simulink model "P_CGMRES_fast"  (R2023a)
settings: Solver=FixedStepAuto  StartTime=0.0  StopTime=22.16  RelTol=1e-3
values from neighbouring files (symbols this model uses):
  lujing = 8    [main.m]
libraries: Solver_SF x1
(part 1 of 21)
settings Model: Creator=Administrator  LastModifiedBy=Lenovo
settings SolverCC: AlgebraicLoopSolver=TrustRegion
settings OptimizationCC: LifeSpan=inf
settings DebuggingCC: UnconnectedInputMsg=warning  UnconnectedOutputMsg=warning  UnconnectedLineMsg=warning  ArithmeticOperatorsInVariantConditions=warning
settings ModelReferenceCC: EnableRefExpFcnMdlSchedulingChecks=on
settings SFSimCC: CustomCodeUndefinedFunction=UseInterfaceOnly
settings CodeAppCC: StateflowObjectComments=on

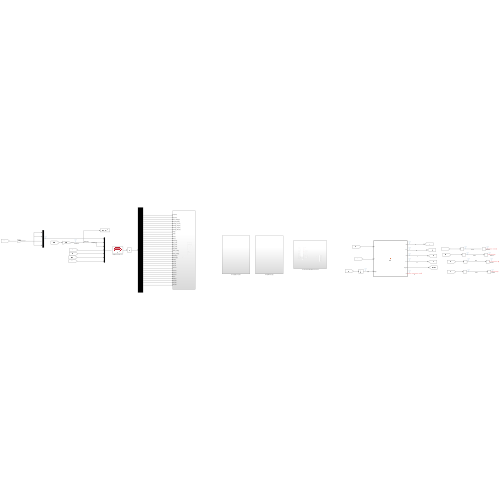
[thumbnail: Simulink's stored preview of the top-level diagram]
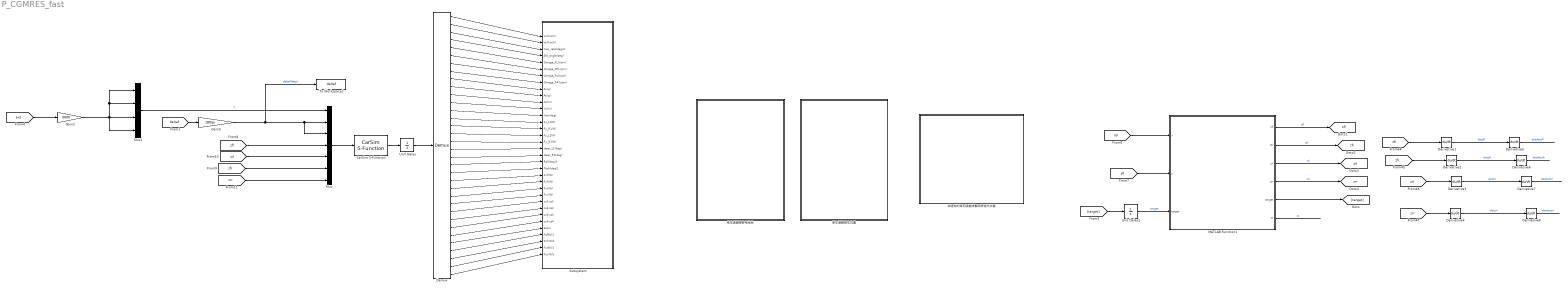
== system P_CGMRES_fast ==
  CarSim S-Function : Solver_SF/CarSim S-Function  Priority=1  SIMFILE=simfile.sim  Run_RTs=off  vs_state_ind=Run  StopMode_ind=Vehicle Model
  Demux : Demux  Outputs=34
  Derivative{1..8} (8 alike) : Derivative
  Gain2 : Gain  Gain=3000
  Gain3 : Gain  Gain=180/pi
  MATLAB Function1 : MATLAB Function  TreatAsAtomicUnit=on
  Mux : Mux  Inputs=7
  Mux1 : Mux
  Subsystem : Subsystem
  To Workspace2 : ToWorkspace  VariableName=deltaf  SaveFormat=Timeseries  SampleTime=-1
  Unit Delay : UnitDelay  InitialCondition=[50,0.01*ones(1,24),0,0,0,0,0,3575,3575,3575,3575]  SampleTime=-1  HasFrameUpgradeWarning=on
  Unit Delay1 : UnitDelay  InitialCondition=1  SampleTime=-1  HasFrameUpgradeWarning=on
  单车道避障参考坐标 : Subsystem
  单车道障碍车位置 : Subsystem
  快速有约束罚函数求解同样迭代次数 : Subsystem
  tag scope: zfl=global, zfr=global, zrl=global, zrr=global
  wires:
  Unit Delay/1 -> Demux/1
  Demux/1 -> Subsystem/1(Vx(km/h))
  Demux/2 -> Subsystem/2(Vy(km/h))
  Demux/3 -> Subsystem/3(Yaw_rate(deg/s))
  Demux/4 -> Subsystem/4(SW_angle(deg))
  Demux/5 -> Subsystem/5(Omega_FL(r/pm))
  Demux/6 -> Subsystem/6(Omega_FR(r/pm))
  Demux/7 -> Subsystem/7(Omega_RL(r/pm))
  Demux/8 -> Subsystem/8(Omega_RR(r/pm))
  Demux/9 -> Subsystem/9(Ax(g))
  Demux/10 -> Subsystem/10(Ay(g))
  Demux/11 -> Subsystem/11(Xo(m))
  Demux/12 -> Subsystem/12(Yo(m))
  Demux/13 -> Subsystem/13(Yaw(deg))
  Demux/14 -> Subsystem/14(Fy_L1(N))
  Demux/15 -> Subsystem/15(Fy_R1(N))
  Demux/16 -> Subsystem/16(Fy_L2(N))
  Demux/17 -> Subsystem/17(Fy_R2(N))
  Demux/18 -> Subsystem/18(steer_L1(deg))
  Demux/19 -> Subsystem/19(steer_R1(deg))
  Mux/1 -> CarSim S-Function/1
  CarSim S-Function/1 -> Unit Delay/1
  [ax2] -> Gain2/1
  Gain2/1 -> Mux1/4, Mux1/3, Mux1/2, Mux1/1
  Mux1/1 -> Mux/1  "T"
  [deltaf] -> Gain3/1
  [zfl] -> Mux/4
  Demux/20 -> Subsystem/20(Roll(deg)1)
  Demux/21 -> Subsystem/21(Pitch(deg)1)
  [zrl] -> Mux/5
  [zfr] -> Mux/6
  [zrr] -> Mux/7
  Demux/22 -> Subsystem/22(Fxfl(N))
  Demux/23 -> Subsystem/23(Fxfr(N))
  Demux/24 -> Subsystem/24(Fxrl(N))
  Demux/25 -> Subsystem/25(Fxrr(N))
  Demux/26 -> Subsystem/26(zu1-zs1)
  Demux/27 -> Subsystem/27(zu2-zs2)
  Demux/28 -> Subsystem/28(zu3-zs3)
  Demux/29 -> Subsystem/29(zu4-zs4)
  Demux/30 -> Subsystem/30(azsm)
  Demux/31 -> Subsystem/31(Fzfl(N)1)
  Demux/32 -> Subsystem/32(Fzfr(N)1)
  Demux/33 -> Subsystem/33(Fzrl(N)1)
  Demux/34 -> Subsystem/34(Fzrr(N)1)
  MATLAB Function1/3(zrl) -> [zrl]  "zrl"
  [zfr] -> Derivative2/1
  Derivative2/1 -> Derivative6/1  "dotzfr"
  Unit Delay1/1 -> MATLAB Function1/3("target ")  "target"
  [target] -> Unit Delay1/1
  [y0] -> MATLAB Function1/2(y)
  [zrr] -> Derivative4/1
  [zfl] -> Derivative1/1
  MATLAB Function1/1(zfl) -> [zfl]  "zfl"
  Derivative1/1 -> Derivative5/1  "dotzfl"
  [zrl] -> Derivative3/1
  Derivative4/1 -> Derivative8/1  "dotzrr"
  MATLAB Function1/4(zrr) -> [zrr]  "zrr"
  [x0] -> MATLAB Function1/1(x)
  MATLAB Function1/5(target) -> [target]
  Derivative3/1 -> Derivative7/1  "dotzrl"
  Derivative6/1 -> ?  "dotdotzfr"
  MATLAB Function1/2(zfr) -> [zfr]  "zfr"
  Derivative5/1 -> ?  "dotdotzfl"
  MATLAB Function1/6(zz) -> ?  "zz"
  Derivative8/1 -> ?  "dotdotzrr"
  Derivative7/1 -> ?  "dotdotzrl"
  Gain3/1 -> To Workspace2/1, Mux/3, Mux/2  "deltaf(deg)"

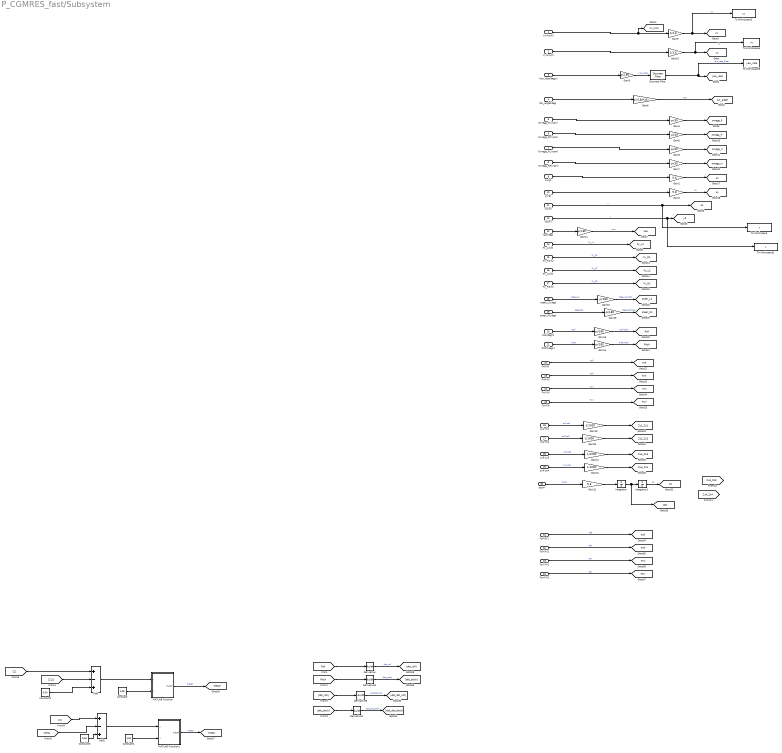
== system P_CGMRES_fast/Subsystem ==
  Vx(km/h) : Inport
  Vy(km/h) : Inport  Port=2
  Yaw_rate(deg/s) : Inport  Port=3
  SW_angle(deg) : Inport  Port=4
  Omega_FL(r/pm) : Inport  Port=5
  Omega_FR(r/pm) : Inport  Port=6
  Omega_RL(r/pm) : Inport  Port=7
  Omega_RR(r/pm) : Inport  Port=8
  Ax(g) : Inport  Port=9
  Ay(g) : Inport  Port=10
  Xo(m) : Inport  Port=11
  Yo(m) : Inport  Port=12
  Yaw(deg) : Inport  Port=13
  Fy_L1(N) : Inport  Port=14
  Fy_R1(N) : Inport  Port=15
  Fy_L2(N) : Inport  Port=16
  Fy_R2(N) : Inport  Port=17
  steer_L1(deg) : Inport  Port=18
  steer_R1(deg) : Inport  Port=19
  Roll(deg)1 : Inport  Port=20
  Pitch(deg)1 : Inport  Port=21
  Fxfl(N) : Inport  Port=22
  Fxfr(N) : Inport  Port=23
  Fxrl(N) : Inport  Port=24
  Fxrr(N) : Inport  Port=25
  zu1-zs1 : Inport  Port=26
  zu2-zs2 : Inport  Port=27
  zu3-zs3 : Inport  Port=28
  zu4-zs4 : Inport  Port=29
  azsm : Inport  Port=30
  Fzfl(N)1 : Inport  Port=31
  Fzfr(N)1 : Inport  Port=32
  Fzrl(N)1 : Inport  Port=33
  Fzrr(N)1 : Inport  Port=34
  Add : Sum  Inputs=+-+
  Add1 : Sum  Inputs=+-+
  Constant : Constant  Value=1.05
  Constant1 : Constant  Value=1.61
  Constant2 : Constant  Value=0.54
  Constant3 : Constant  Value=0.54
  Derivative{,1..3} (4 alike) : Derivative
  Discrete Filter : DiscreteFilter
  Gain1 : Gain  Gain=9.8
  Gain10 : Gain  Gain=1/3.6
  Gain{3,11,13..16} (6 alike) : Gain  Gain=pi/180
  Gain12 : Gain  Gain=9.8
  Gain{19..22} (4 alike) : Gain  Gain=1/1000
  Gain2 : Gain  Gain=9.8
  Gain{4..7} (4 alike) : Gain  Gain=pi/30
  Gain8 : Gain  Gain=pi/(180*16)
  Gain9 : Gain  Gain=1/3.6
  Integrator : Integrator
  Integrator1 : Integrator  InitialCondition=0.54
  MATLAB Function : MATLAB Function  TreatAsAtomicUnit=on
  MATLAB Function1 : MATLAB Function  TreatAsAtomicUnit=on
  To Workspace : ToWorkspace  VariableName=x  SaveFormat=Timeseries  SampleTime=-1
  To Workspace1 : ToWorkspace  VariableName=y  SaveFormat=Timeseries  SampleTime=-1
  To Workspace2 : ToWorkspace  VariableName=vx  SaveFormat=Timeseries  SampleTime=-1
  To Workspace3 : ToWorkspace  VariableName=yaw_rate  SampleTime=-1
      settings: Save2DSignal=2-D array (concatenate along first dimension)
  To Workspace4 : ToWorkspace  VariableName=Vy  SampleTime=-1
      settings: Save2DSignal=2-D array (concatenate along first dimension)
  tag scope: Fxfl=global, Fxfr=global, Fxrl=global, Fxrr=global, Fy_L1=global, Fy_L2=global, Fy_R1=global, Fy_R2=global, Fzfl=global, Fzfr=global, Fzrl=global, Fzrr=global, Pitch=global, Roll=global, Vx=global, Vx_kmh=global, Vy=global, Yaw=global, Zs=global, Zu1_Zs1=global, Zu2_Zs2=global, Zu3_Zs3=global, Zu4_Zs4=global, ax=global, ay=global, dZs=global, omega_fl=global, omega_fr=global, omega_rl=global, omega_rr=global, steer_L1=global, steer_R1=global, sw_angle=global, thetaf=global, thetar=global, x0=global, y0=global, yaw_rate=global
  wires:
  Vy(km/h)/1 -> Gain10/1
  Gain4/1 -> [omega_fl]
  Ay(g)/1 -> Gain2/1
  Gain6/1 -> [omega_rl]
  Gain7/1 -> [omega_rr]
  Gain10/1 -> To Workspace4/1, [Vy]  "Vy"
  Gain1/1 -> [ax]
  Gain3/1 -> Discrete Filter/1  "yaw_rate"
  Yaw_rate(deg/s)/1 -> Gain3/1
  Gain5/1 -> [omega_fr]
  Gain8/1 -> [sw_angle]  "SW"
  Gain2/1 -> [ay]  "ay"
  Vx(km/h)/1 -> [Vx_kmh], Gain9/1
  Omega_RR(r/pm)/1 -> Gain7/1
  Omega_FR(r/pm)/1 -> Gain5/1
  Omega_RL(r/pm)/1 -> Gain6/1
  Ax(g)/1 -> Gain1/1
  SW_angle(deg)/1 -> Gain8/1
  Omega_FL(r/pm)/1 -> Gain4/1
  Yaw(deg)/1 -> Gain11/1
  Gain11/1 -> [Yaw]  "yaw"
  Fy_L1(N)/1 -> [Fy_L1]  "Fy_L1"
  Fy_R1(N)/1 -> [Fy_R1]  "Fy_R1"
  Fy_L2(N)/1 -> [Fy_L2]  "Fy_L2"
  Fy_R2(N)/1 -> [Fy_R2]  "Fy_R2"
  steer_L1(deg)/1 -> Gain15/1  "steer_L1"
  steer_R1(deg)/1 -> Gain16/1  "steer_R1"
  Discrete Filter/1 -> [yaw_rate], To Workspace3/1  "yaw_rate_filter"
  Roll(deg)1/1 -> Gain13/1  "Roll"
  Pitch(deg)1/1 -> Gain14/1  "Pitch"
  Fxfr(N)/1 -> [Fxfr]  "Fxfr"
  Fxfl(N)/1 -> [Fxfl]  "Fxfl"
  Fxrr(N)/1 -> [Fxrr]  "Fxrr"
  Fxrl(N)/1 -> [Fxrl]  "Fxrl"
  Gain13/1 -> [Roll]  "Roll(rad)"
  Gain14/1 -> [Pitch]  "Pitch(rad)"
  Gain15/1 -> [steer_L1]  "steer_L1(rad)"
  Gain16/1 -> [steer_R1]  "steer_R1(rad)"
  [Roll] -> Derivative/1
  [Pitch] -> Derivative1/1
  Derivative/1 -> [dot_roll]  "dot_roll"
  Derivative1/1 -> [dot_pitch]  "dot_pitch"
  [dot_roll] -> Derivative3/1
  [dot_pitch] -> Derivative2/1
  Derivative3/1 -> [dot_dot_roll]  "dot_dot_roll"
  Derivative2/1 -> [dot_dot_pitch]  "dot_dot_pitch"
  [Z] -> Add/1
  [ZL1] -> Add/2
  Add/1 -> MATLAB Function/1(y)
  MATLAB Function/1(thetaf) -> [thetaf]  "thetaf"
  Constant/1 -> MATLAB Function/2(x)
  [Z] -> Add1/1
  Add1/1 -> MATLAB Function1/1(y)
  [ZR1] -> Add1/2
  Constant1/1 -> MATLAB Function1/2(x)
  MATLAB Function1/1(thetaf) -> [thetar]  "thetar"
  Constant2/1 -> Add/3
  Constant3/1 -> Add1/3
  zu1-zs1/1 -> Gain19/1  "zu1-zs1"
  zu3-zs3/1 -> Gain21/1  "zu3-zs3"
  Gain19/1 -> [Zu1_Zs1]
  Gain21/1 -> [Zu3_Zs3]
  zu2-zs2/1 -> Gain20/1  "zu2-zs2"
  Gain22/1 -> [Zu4_Zs4]
  Gain20/1 -> [Zu2_Zs2]
  zu4-zs4/1 -> Gain22/1  "zu4-zs4"
  azsm/1 -> Gain12/1  "azsm"
  Gain12/1 -> Integrator/1
  Integrator/1 -> [dZs], Integrator1/1
  Integrator1/1 -> [Zs]  "zs"
  Fzfl(N)1/1 -> [Fzfl]  "Fzfl"
  Fzrl(N)1/1 -> [Fzrl]  "Fzrl"
  Fzfr(N)1/1 -> [Fzfr]  "Fzfr"
  Fzrr(N)1/1 -> [Fzrr]  "Fzrr"
  Gain9/1 -> To Workspace2/1, [Vx]  "Vx"
  Xo(m)/1 -> To Workspace/1, [x0]  "x"
  Yo(m)/1 -> To Workspace1/1, [y0]  "y"

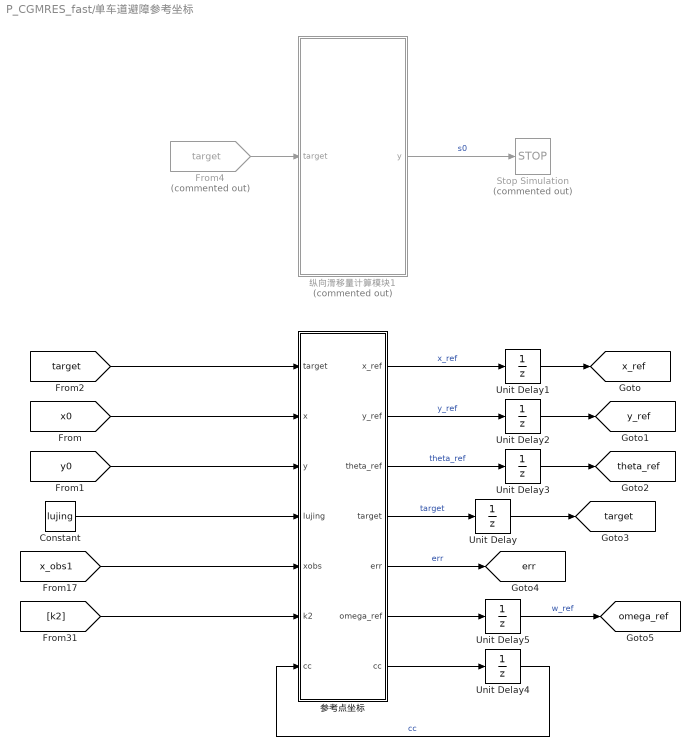
== system P_CGMRES_fast/单车道避障参考坐标 ==
  Constant : Constant  Value=lujing
  From4 : From  Commented=on  GotoTag=target  TagVisibility=global
  Stop Simulation : Stop  Commented=on
  Unit Delay : UnitDelay  InitialCondition=1  SampleTime=-1  HasFrameUpgradeWarning=on
  Unit Delay{1..3,5} (4 alike) : UnitDelay  InitialCondition=ones(10,1)*0  SampleTime=-1  HasFrameUpgradeWarning=on
  Unit Delay4 : UnitDelay  SampleTime=-1  HasFrameUpgradeWarning=on
  参考点坐标 : MATLAB Function  TreatAsAtomicUnit=on
  纵向滑移量计算模块1 : MATLAB Function  Commented=on  TreatAsAtomicUnit=on
  tag scope: err=global, omega_ref=global, target=global, theta_ref=global, x_ref=global, y_ref=global
  wires:
  [x0] -> 参考点坐标/2(x)
  [y0] -> 参考点坐标/3(y)
  参考点坐标/2(y_ref) -> Unit Delay2/1  "y_ref"
  参考点坐标/3(theta_ref) -> Unit Delay3/1  "theta_ref"
  参考点坐标/4(target) -> Unit Delay/1  "target"
  参考点坐标/1(x_ref) -> Unit Delay1/1  "x_ref"
  [target] -> 参考点坐标/1("target ")
  Unit Delay/1 -> [target]
  参考点坐标/5(err) -> [err]  "err"
  纵向滑移量计算模块1/1(y) -> Stop Simulation/1  "s0"
  From4/1 -> 纵向滑移量计算模块1/1("target ")
  Unit Delay1/1 -> [x_ref]
  Unit Delay2/1 -> [y_ref]
  Unit Delay3/1 -> [theta_ref]
  Constant/1 -> 参考点坐标/4(lujing)
  参考点坐标/6(omega_ref) -> Unit Delay5/1
  Unit Delay5/1 -> [omega_ref]  "w_ref"
  [x_obs1] -> 参考点坐标/5(xobs)
  [k2] -> 参考点坐标/6(k2)
  参考点坐标/7(cc) -> Unit Delay4/1
  Unit Delay4/1 -> 参考点坐标/7("cc ")  "cc"

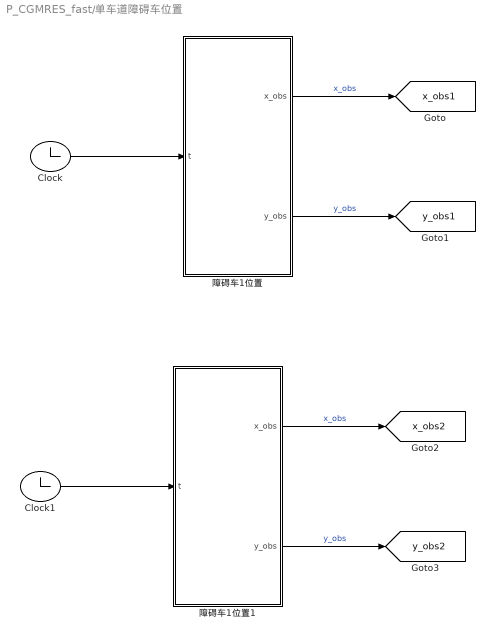
== system P_CGMRES_fast/单车道障碍车位置 ==
  Clock : Clock
  Clock1 : Clock
  障碍车1位置 : MATLAB Function  TreatAsAtomicUnit=on
  障碍车1位置1 : MATLAB Function  TreatAsAtomicUnit=on
  tag scope: x_obs1=global, x_obs2=global, y_obs1=global, y_obs2=global
  wires:
  障碍车1位置/1(x_obs) -> [x_obs1]  "x_obs"
  障碍车1位置/2(y_obs) -> [y_obs1]  "y_obs"
  Clock/1 -> 障碍车1位置/1(t)
  Clock1/1 -> 障碍车1位置1/1(t)
  障碍车1位置1/1(x_obs) -> [x_obs2]  "x_obs"
  障碍车1位置1/2(y_obs) -> [y_obs2]  "y_obs"

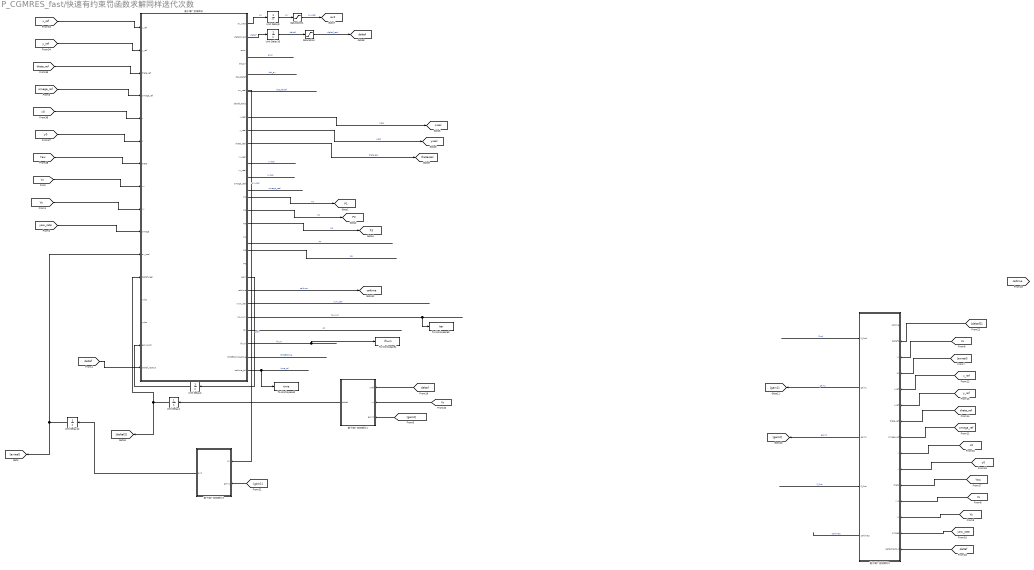
== system P_CGMRES_fast/快速有约束罚函数求解同样迭代次数 ==
  Saturation : Saturate  UpperLimit=0.2  LowerLimit=-0.2
  Saturation1 : Saturate  UpperLimit=0.05  LowerLimit=-0.05
  To Workspace1 : ToWorkspace  VariableName=ifnum  SaveFormat=Timeseries  SampleTime=-1
  To Workspace2 : ToWorkspace  VariableName=time  SaveFormat=Timeseries  SampleTime=-1
  To Workspace3 : ToWorkspace  VariableName=iter  SaveFormat=Timeseries  SampleTime=-1
  Unit Delay1 : UnitDelay  InitialCondition=ones(10,1)*0  SampleTime=-1  HasFrameUpgradeWarning=on
  Unit Delay10 : UnitDelay  SampleTime=-1  HasFrameUpgradeWarning=on
  Unit Delay12 : UnitDelay  InitialCondition=ones(10,1)  SampleTime=-1  HasFrameUpgradeWarning=on
  Unit Delay2 : UnitDelay  SampleTime=-1  HasFrameUpgradeWarning=on
  Unit Delay9 : UnitDelay  SampleTime=-1  HasFrameUpgradeWarning=on
  基于增广拉格朗日 : MATLAB Function  TreatAsAtomicUnit=on
  基于增广拉格朗日1 : MATLAB Function  TreatAsAtomicUnit=on
  基于增广拉格朗日2 : MATLAB Function  TreatAsAtomicUnit=on
  基于增广拉格朗日3 : MATLAB Function  TreatAsAtomicUnit=on
  tag scope: P1=global, P2=global, P3=global, ax2=global, caltime=global, deltaf=global, thetareal=global, xreal=global, yreal=global
  wires:
  [Yaw] -> 基于增广拉格朗日/7(theta)
  [y0] -> 基于增广拉格朗日/6(y)
  [x0] -> 基于增广拉格朗日/5(x)
  [y_ref] -> 基于增广拉格朗日/2(y_ref)
  [omega_ref] -> 基于增广拉格朗日/4(omega_ref)
  [x_ref] -> 基于增广拉格朗日/1(x_ref)
  [theta_ref] -> 基于增广拉格朗日/3(theta_ref)
  基于增广拉格朗日/1(ax_next) -> Unit Delay9/1  "ax"
  基于增广拉格朗日/2(deltaf_next) -> Unit Delay10/1  "deltaf"
  基于增广拉格朗日/3(error) -> ?  "error"
  基于增广拉格朗日/6(ax_real) -> 基于增广拉格朗日3/1(ax)  "ax_real"
  基于增广拉格朗日/13(omega_real) -> ?  "omega_real"
  基于增广拉格朗日/15(P2) -> [P2]  "P2"
  基于增广拉格朗日/14(P1) -> [P1]  "P1"
  基于增广拉格朗日/16(P3) -> [P3]  "P3"
  基于增广拉格朗日/8(x_real) -> [xreal]  "xreal"
  基于增广拉格朗日/9(y_real) -> [yreal]  "yreal"
  基于增广拉格朗日/10(theta_real) -> [thetareal]  "thetareal"
  基于增广拉格朗日/4(dot_ax) -> ?  "dot_ax"
  基于增广拉格朗日/5(dot_deltaf) -> ?  "dot_deltaf"
  基于增广拉格朗日/11(vx_real) -> ?  "vxreal"
  基于增广拉格朗日/12(vy_real) -> ?  "vyreal"
  基于增广拉格朗日/17(P4) -> ?  "P4"
  基于增广拉格朗日/18(P5) -> ?  "P5"
  Unit Delay12/1 -> [axreal], 基于增广拉格朗日/11("ax_real ")
  [Vx] -> 基于增广拉格朗日/8(vx)
  [Vy] -> 基于增广拉格朗日/9(vy)
  [yaw_rate] -> 基于增广拉格朗日/10(omega)
  Unit Delay9/1 -> Saturation1/1  "ax"
  Unit Delay10/1 -> Saturation/1  "deltaf"
  Unit Delay1/1 -> [deltaf2], 基于增广拉格朗日/12(deltaf_real)
  基于增广拉格朗日/20(gain) -> Unit Delay2/1  "gain"
  Unit Delay2/1 -> 基于增广拉格朗日/15(gain_last)
  基于增广拉格朗日/21(caltime) -> [caltime]  "caltime"
  [Vx] -> 基于增广拉格朗日2/3(vx)
  Saturation/1 -> [deltaf]  "deltaf_real"
  Saturation1/1 -> [ax2]  "ax_real"
  [deltaf] -> 基于增广拉格朗日/16(deltaf_lastout)
  基于增广拉格朗日/22(num_iter) -> ?  "num_iter"
  [deltaf2] -> 基于增广拉格朗日2/2(deltaf2)
  [axreal] -> 基于增广拉格朗日2/4(ax)
  [x_ref] -> 基于增广拉格朗日2/5(x_ref)
  [y_ref] -> 基于增广拉格朗日2/6(y_ref)
  [theta_ref] -> 基于增广拉格朗日2/7(theta_ref)
  [omega_ref] -> 基于增广拉格朗日2/8(omega_ref)
  [x0] -> 基于增广拉格朗日2/9(x)
  [y0] -> 基于增广拉格朗日2/10(y)
  [Yaw] -> 基于增广拉格朗日2/11(theta)
  [Vx] -> 基于增广拉格朗日2/12(vx1)
  [Vy] -> 基于增广拉格朗日2/13(vy)
  [yaw_rate] -> 基于增广拉格朗日2/14(omega)
  [deltaf] -> 基于增广拉格朗日2/15(deltaf_lastout)
  基于增广拉格朗日1/1(deltaf) -> Unit Delay1/1
  [deltaf] -> 基于增广拉格朗日1/1(wref)
  [Vx] -> 基于增广拉格朗日1/2(vx)
  基于增广拉格朗日2/2(gain1) -> [gain1]  "gain1"
  基于增广拉格朗日2/3(gain2) -> [gain2]  "gain2"
  基于增广拉格朗日2/4(F_first) -> ?  "F_first"
  基于增广拉格朗日/24(FF) -> ?  "FF"
  基于增广拉格朗日2/1(F_final) -> ?  "Final"
  [gain2] -> 基于增广拉格朗日1/3(gain2)
  基于增广拉格朗日3/1(ax2) -> Unit Delay12/1
  [gain1] -> 基于增广拉格朗日3/2(gain1)
  基于增广拉格朗日2/5(caltime2) -> ?  "caltime2"
  基于增广拉格朗日/26(GMRESsimpletime) -> ?  "GMREStime"
  基于增广拉格朗日/27(caltime_tol) -> To Workspace2/1  "time_tol"
  基于增广拉格朗日/25(ifnum) -> To Workspace1/1  "ifnum"
  基于增广拉格朗日/23(kp_num) -> To Workspace3/1  "kp_num"
